simulink model "StateMachine"  (R2024a)
settings: Solver=ode4  StartTime=0.0  StopTime=10.0  FixedStep=1/1600  RelTol=1e-3
undefined symbols (not defined in the file): gains, initout, params, rates
libraries: simulink_extras x4, slpidlib x2, GT x1, aerolibasang x1
settings Model: Creator=igmso  LastModifiedBy=igmso

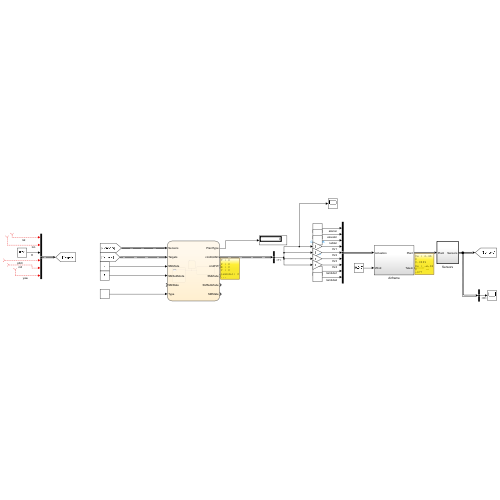
[thumbnail: Simulink's stored preview of the top-level diagram]
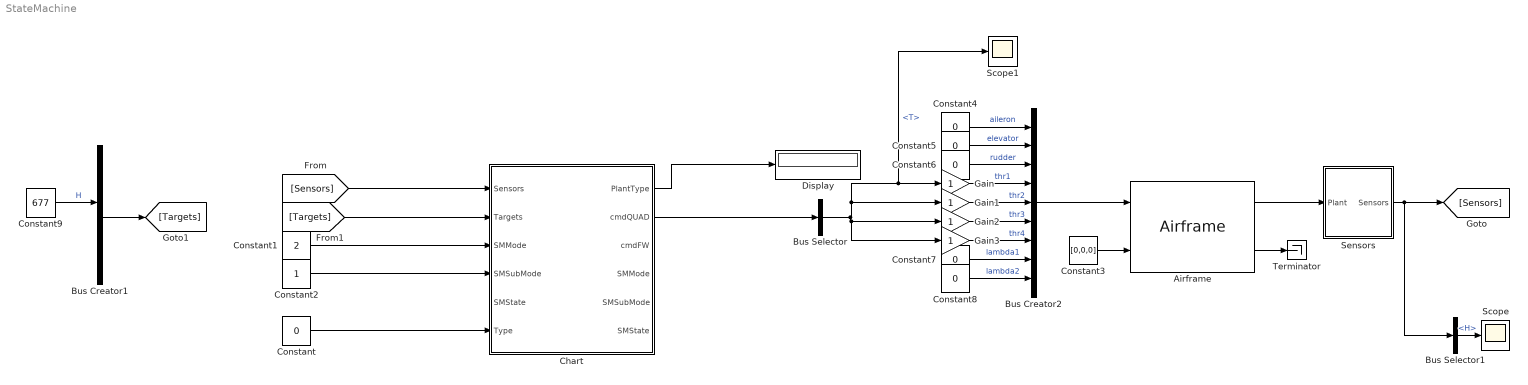
== system StateMachine ==
  Airframe : GT/Airframe  SystemSampleTime=-1  VariantActivationTime=update diagram  AllowFlexibleInterface=on  Latency=0  AutoFrameSizeCalculation=off
  Bus Creator1 : BusCreator  Inputs=6  OutDataTypeStr=Bus: targetsBus  NonVirtualBus=on
  Bus Creator2 : BusCreator  Inputs=9
  Bus Selector : BusSelector  OutputSignals=T
  Bus Selector1 : BusSelector  OutputSignals=H
  Chart : Stateflow chart  TreatAsAtomicUnit=on
      settings: PortSchema="{\"entries\":[{\"content\":{\"sides\":[{\"content\":{\"connectorIds\":[\"In1\",\"In2\",\"In3\",\"In4\",\"In5\",\"In6\"]},\"type\":\"ConnectorPlacement.EquallySpacedRectSide\",\"uuid\":\"c12811fb-1763-4b1f-8237-72373105f559\"},{\"content\":{\"connectorIds\":[\"Out1\",\"Out5\",\"Out6\",\"Out2\",\"Out3\",\"Out4\"],\"side\":\"RIGHT\"},\"type\":\"ConnectorPlacement.EquallySpacedRectSide\",\"uuid\":\"3712ff0d-cc13-4e2e-bfea-d52da842e5af\"},{\"content\":{\"side\":\"TOP\"},\"type\":\"ConnectorPlacement.EquallySpacedRectSide\",\"uuid\":\"ba161a25-7347-4103-889e-23a821fde0ef\"}]},\"type\":\"ConnectorPlacement.EquallySpacedConnector\",\"uuid\":\"8d874a7a-8fc0-4a11-bc61-1ae99cb768d4\"}],\"packageUris\":[\"http://schema.mathworks.com/mf0/Connector/R2020b\"],\"version\":\"1.0\"}"
  Constant{,4..8} (6 alike) : Constant  Value=0  SampleTime=-1
  Constant1 : Constant  Value=2  SampleTime=-1
  Constant2 : Constant  SampleTime=-1
  Constant3 : Constant  Value=[0,0,0]  SampleTime=-1
  Constant9 : Constant  Value=677  SampleTime=-1
  Display : Display
  Gain{,1..3} (4 alike) : Gain
  Scope : Scope
  Scope1 : Scope
  Sensors : Subsystem  TreatAsAtomicUnit=on  SystemSampleTime=1/400
  Terminator : Terminator
  wires:
  Constant/1 -> Chart/6(Type)
  Chart/1(PlantType) -> Display/1
  [Sensors] -> Chart/1(Sensors)
  Bus Creator1/1 -> [Targets]
  Constant9/1 -> Bus Creator1/3  "H"
  [Targets] -> Chart/2(Targets)
  Constant1/1 -> Chart/3("SMMode ")
  Constant2/1 -> Chart/4("SMSubMode ")
  Airframe/1 -> Sensors/1(Plant)
  Sensors/1(Sensors) -> Bus Selector1/1, [Sensors]
  Airframe/2 -> Terminator/1
  Constant3/1 -> Airframe/2
  Gain2/1 -> Bus Creator2/6  "thr3"
  Constant4/1 -> Bus Creator2/1  "aileron"
  Gain1/1 -> Bus Creator2/5  "thr2"
  Constant6/1 -> Bus Creator2/3  "rudder"
  Gain/1 -> Bus Creator2/4  "thr1"
  Constant8/1 -> Bus Creator2/9  "lambda2"
  Gain3/1 -> Bus Creator2/7  "thr4"
  Constant7/1 -> Bus Creator2/8  "lambda1"
  Constant5/1 -> Bus Creator2/2  "elevator"
  Bus Creator2/1 -> Airframe/1
  Chart/5(cmdQUAD) -> Bus Selector/1
  Bus Selector/1 -> Gain3/1, Gain2/1, Gain1/1, Scope1/1, Gain/1  "<T>"
  ? -> Bus Creator1/1  "lat"
  ? -> Bus Creator1/2  "lon"
  ? -> Bus Creator1/4  "pitch"
  ? -> Bus Creator1/5  "roll"
  ? -> Bus Creator1/6  "yaw"
  Bus Selector1/1 -> Scope/1  "<H>"

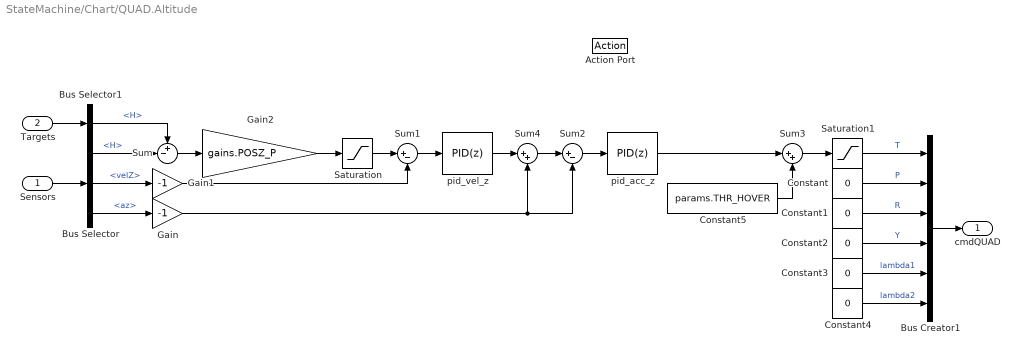
== system StateMachine/Chart/QUAD.Altitude ==
  Sensors : Inport  OutDataTypeStr=Bus: sensorsBus
  Targets : Inport  Port=2  OutDataTypeStr=Bus: targetsBus
  Action Port : ActionPort
      settings: CopyFcn=Stateflow.SLINSF.SimulinkMan.removeBlockPreDeleteFcn  PreDeleteFcn=Stateflow.SLINSF.SimulinkMan.unsafePredeleteFcn
  Bus Creator1 : BusCreator  Inputs=6  OutDataTypeStr=Bus: cmdQUADBus  NonVirtualBus=on
  Bus Selector : BusSelector  OutputSignals=H,velZ,az
  Bus Selector1 : BusSelector  OutputSignals=H
  Constant{,1..4} (5 alike) : Constant  Value=0  SampleTime=-1
  Constant5 : Constant  Value=params.THR_HOVER
  Gain : Gain  Gain=-1
  Gain1 : Gain  Gain=-1
  Gain2 : Gain  Gain=gains.POSZ_P
  Saturation : Saturate  UpperLimit=1  LowerLimit=-1
  Saturation1 : Saturate  UpperLimit=1  LowerLimit=0
  Sum : Sum  Inputs=+-|
  Sum1 : Sum  Inputs=|+-
  Sum2 : Sum  Inputs=|+-
  Sum3 : Sum  Inputs=|++
  Sum4 : Sum  Inputs=|++
  pid_acc_z : slpidlib/PID Controller  Controller=PID  Form=Parallel  TimeDomain=Discrete-time  UseExternalTs=off  SampleTime=rates.Altitude  IntegratorMethod=Forward Euler  FilterMethod=Forward Euler  ControllerParametersSource=internal  P=gains.ACCZ_P  I=gains.ACCZ_I  UseKiTs=on  D=gains.ACCZ_D  UseExternalDerivativeSource=off  N=gains.ACCZ_FF  UseFilter=on  TunerSelectOption=Transfer Function Based (PID Tuner App)  InitialConditionSource=internal  InitialConditionForIntegrator=0  InitialConditionForFilter=0  DifferentiatorICPrevScaledInput=0  ExternalReset=none  TrackingMode=off  Kt=1  LimitOutput=off  SatLimitsSource=internal  UpperSaturationLimit=params.CLIMB_MAX  LowerSaturationLimit=-params.SINK_MAX  LinearizeAsGain=on  AntiWindupMode=clamping  Kb=1  LimitIntegrator=on  UpperIntegratorSaturationLimit=gains.VELZ_IMAX  LowerIntegratorSaturationLimit=-gains.VELZ_IMAX  POutMin=[]  POutMax=[]  IOutMin=[]  IOutMax=[]  DOutMin=[]  DOutMax=[]  NOutMin=[]  NOutMax=[]  SumOutMin=[]  SumOutMax=[]  SaturationOutMin=[]  SaturationOutMax=[]  PParamMin=[]  PParamMax=[]  IParamMin=[]  IParamMax=[]  DParamMin=[]  DParamMax=[]  NParamMin=[]  NParamMax=[]  KbParamMin=[]  KbParamMax=[]  KtParamMin=[]  KtParamMax=[]  KbOutMin=[]  KbOutMax=[]  KtOutMin=[]  KtOutMax=[]  IntegratorOutMin=[]  IntegratorOutMax=[]  FilterOutMin=[]  FilterOutMax=[]  SumI1OutMin=[]  SumI1OutMax=[]  SumI2OutMin=[]  SumI2OutMax=[]  SumI3OutMin=[]  SumI3OutMax=[]  SumI4OutMin=[]  SumI4OutMax=[]  SumDOutMin=[]  SumDOutMax=[]  DifferentiatorOutMin=[]  DifferentiatorOutMax=[]  FilterDiffOutCoefMin=[]  FilterDiffOutCoefMax=[]  ReciprocalOutMin=[]  ReciprocalOutMax=[]  SumDenOutMin=[]  SumDenOutMax=[]  SumNumOutMin=[]  SumNumOutMax=[]  DivideOutMin=[]  DivideOutMax=[]  UdiffTsProdOutMin=[]  UdiffTsProdOutMax=[]  NTsProdOutMin=[]  NTsProdOutMax=[]  UintegralTsProdOutMin=[]  UintegralTsProdOutMax=[]  UngainTsProdOutMin=[]  UngainTsProdOutMax=[]  ClampingZeroOutDataTypeStr=Inherit: Inherit via back propagation  ClampingZeroOutMin=[]  ClampingZeroOutMax=[]  FilterDenConstantOutDataTypeStr=Inherit: Inherit via back propagation  FilterDenConstantOutMin=[]  FilterDenConstantOutMax=[]  PCopyOutDataTypeStr=Inherit: Inherit via back propagation  PCopyOutMin=[]  PCopyOutMax=[]  NCopyOutDataTypeStr=Inherit: Inherit via back propagation  NCopyOutMin=[]  NCopyOutMax=[]  IntegratorContinuousStateAttributes=''  IntegratorStateIdentifier="\"VELZ\""  IntegratorStateMustResolveToSignalObject=off  IntegratorRTWStateStorageClass=Auto  FilterContinuousStateAttributes=''  FilterStateIdentifier="\"VELZ\""  FilterStateMustResolveToSignalObject=off  FilterRTWStateStorageClass=Auto  ParallelPVariant=InternalParameters  IdealPVariant=Disabled  IVariant=InternalParameters  DVariant=InternalParameters  IntegratorVariant=Discrete  SatVariant=Disabled  AWVariant=Passthrough  PCopyVariant=Disabled  TRVariant=Disabled  FdbkBlocksVariant=Forward  IdealPFdbkVariant=Disabled  SatFdbkVariant=Disabled  DerivativeFilterVariant=ForwardEulerFilter  NVariant=InternalParameters  NCopyVariant=Disabled  FilterICVariant=InternalICsFilter  IntegratorICVariant=InternalICs  ExternalResetVariant=Disabled  TRSumVariant=Passthrough  SumFdbkVariant=Disabled  SumVariant=Sum_PID  TsampFilterVariant=InternalTs  TsampNgainVariant=Passthrough  TsampIntegralVariant=Disabled_SignalSpec  ExternalSaturationOutDataTypeStr=Inherit: Same as second input  DerivativeSourceVariant=ErrorSignal
  pid_vel_z : slpidlib/PID Controller  Controller=PID  Form=Parallel  TimeDomain=Discrete-time  UseExternalTs=off  SampleTime=rates.Altitude  IntegratorMethod=Forward Euler  FilterMethod=Forward Euler  ControllerParametersSource=internal  P=gains.VELZ_P  I=gains.VELZ_I  UseKiTs=on  D=gains.VELZ_D  UseExternalDerivativeSource=off  N=gains.VELZ_FF  UseFilter=on  TunerSelectOption=Transfer Function Based (PID Tuner App)  InitialConditionSource=internal  InitialConditionForIntegrator=0  InitialConditionForFilter=0  DifferentiatorICPrevScaledInput=0  ExternalReset=none  TrackingMode=off  Kt=1  LimitOutput=off  SatLimitsSource=internal  UpperSaturationLimit=params.CLIMB_MAX  LowerSaturationLimit=-params.SINK_MAX  LinearizeAsGain=on  AntiWindupMode=clamping  Kb=1  LimitIntegrator=on  UpperIntegratorSaturationLimit=gains.VELZ_IMAX  LowerIntegratorSaturationLimit=-gains.VELZ_IMAX  POutMin=[]  POutMax=[]  IOutMin=[]  IOutMax=[]  DOutMin=[]  DOutMax=[]  NOutMin=[]  NOutMax=[]  SumOutMin=[]  SumOutMax=[]  SaturationOutMin=[]  SaturationOutMax=[]  PParamMin=[]  PParamMax=[]  IParamMin=[]  IParamMax=[]  DParamMin=[]  DParamMax=[]  NParamMin=[]  NParamMax=[]  KbParamMin=[]  KbParamMax=[]  KtParamMin=[]  KtParamMax=[]  KbOutMin=[]  KbOutMax=[]  KtOutMin=[]  KtOutMax=[]  IntegratorOutMin=[]  IntegratorOutMax=[]  FilterOutMin=[]  FilterOutMax=[]  SumI1OutMin=[]  SumI1OutMax=[]  SumI2OutMin=[]  SumI2OutMax=[]  SumI3OutMin=[]  SumI3OutMax=[]  SumI4OutMin=[]  SumI4OutMax=[]  SumDOutMin=[]  SumDOutMax=[]  DifferentiatorOutMin=[]  DifferentiatorOutMax=[]  FilterDiffOutCoefMin=[]  FilterDiffOutCoefMax=[]  ReciprocalOutMin=[]  ReciprocalOutMax=[]  SumDenOutMin=[]  SumDenOutMax=[]  SumNumOutMin=[]  SumNumOutMax=[]  DivideOutMin=[]  DivideOutMax=[]  UdiffTsProdOutMin=[]  UdiffTsProdOutMax=[]  NTsProdOutMin=[]  NTsProdOutMax=[]  UintegralTsProdOutMin=[]  UintegralTsProdOutMax=[]  UngainTsProdOutMin=[]  UngainTsProdOutMax=[]  ClampingZeroOutDataTypeStr=Inherit: Inherit via back propagation  ClampingZeroOutMin=[]  ClampingZeroOutMax=[]  FilterDenConstantOutDataTypeStr=Inherit: Inherit via back propagation  FilterDenConstantOutMin=[]  FilterDenConstantOutMax=[]  PCopyOutDataTypeStr=Inherit: Inherit via back propagation  PCopyOutMin=[]  PCopyOutMax=[]  NCopyOutDataTypeStr=Inherit: Inherit via back propagation  NCopyOutMin=[]  NCopyOutMax=[]  IntegratorContinuousStateAttributes=''  IntegratorStateIdentifier="\"VELZ\""  IntegratorStateMustResolveToSignalObject=off  IntegratorRTWStateStorageClass=Auto  FilterContinuousStateAttributes=''  FilterStateIdentifier="\"VELZ\""  FilterStateMustResolveToSignalObject=off  FilterRTWStateStorageClass=Auto  ParallelPVariant=InternalParameters  IdealPVariant=Disabled  IVariant=InternalParameters  DVariant=InternalParameters  IntegratorVariant=Discrete  SatVariant=Disabled  AWVariant=Passthrough  PCopyVariant=Disabled  TRVariant=Disabled  FdbkBlocksVariant=Forward  IdealPFdbkVariant=Disabled  SatFdbkVariant=Disabled  DerivativeFilterVariant=ForwardEulerFilter  NVariant=InternalParameters  NCopyVariant=Disabled  FilterICVariant=InternalICsFilter  IntegratorICVariant=InternalICs  ExternalResetVariant=Disabled  TRSumVariant=Passthrough  SumFdbkVariant=Disabled  SumVariant=Sum_PID  TsampFilterVariant=InternalTs  TsampNgainVariant=Passthrough  TsampIntegralVariant=Disabled_SignalSpec  ExternalSaturationOutDataTypeStr=Inherit: Same as second input  DerivativeSourceVariant=ErrorSignal
  cmdQUAD : Outport  OutDataTypeStr=Bus: cmdQUADBus
  wires:
  Sensors/1 -> Bus Selector/1
  Bus Selector/3 -> Gain/1  "<az>"
  Bus Selector/2 -> Gain1/1  "<velZ>"
  Bus Selector/1 -> Sum/2  "<H>"
  Bus Selector1/1 -> Sum/1  "<H>"
  Targets/1 -> Bus Selector1/1
  Sum/1 -> Gain2/1
  Gain2/1 -> Saturation/1
  Gain1/1 -> Sum1/2
  Sum1/1 -> pid_vel_z/1
  pid_vel_z/1 -> Sum4/1
  Gain/1 -> Sum4/2, Sum2/2
  Sum2/1 -> pid_acc_z/1
  Saturation/1 -> Sum1/1
  Saturation1/1 -> Bus Creator1/1  "T"
  pid_acc_z/1 -> Sum3/1
  Constant/1 -> Bus Creator1/2  "P"
  Constant1/1 -> Bus Creator1/3  "R"
  Constant2/1 -> Bus Creator1/4  "Y"
  Constant3/1 -> Bus Creator1/5  "lambda1"
  Constant4/1 -> Bus Creator1/6  "lambda2"
  Bus Creator1/1 -> cmdQUAD/1
  Sum3/1 -> Saturation1/1
  Constant5/1 -> Sum3/2
  Sum4/1 -> Sum2/1

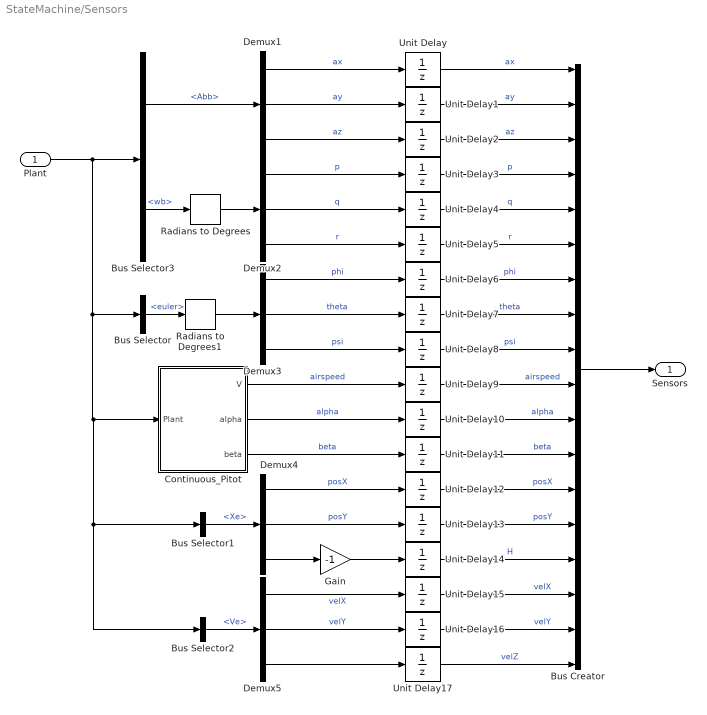
== system StateMachine/Sensors ==
  Plant : Inport
  Bus Selector : BusSelector  OutputSignals=euler
  Bus Selector1 : BusSelector  OutputSignals=Xe
  Bus Selector2 : BusSelector  OutputSignals=Ve
  Bus Selector3 : BusSelector  OutputSignals=Abb,wb
  Bus Creator : BusCreator  Inputs=18  OutDataTypeStr=Bus: sensorsBus  NonVirtualBus=on
  Continuous_Pitot : Subsystem
  Demux{1..5} (5 alike) : Demux  Outputs=3
  Gain : Gain  Gain=-1
  Radians to Degrees : simulink_extras/Transformations/Radians to Degrees
  Radians to Degrees1 : simulink_extras/Transformations/Radians to Degrees
  Unit Delay : UnitDelay  InitialCondition=initout(1)  SampleTime=-1  HasFrameUpgradeWarning=on
  Unit Delay1 : UnitDelay  InitialCondition=initout(2)  SampleTime=-1  HasFrameUpgradeWarning=on
  Unit Delay10 : UnitDelay  InitialCondition=initout(11)  SampleTime=-1  HasFrameUpgradeWarning=on
  Unit Delay11 : UnitDelay  InitialCondition=initout(12)  SampleTime=-1  HasFrameUpgradeWarning=on
  Unit Delay12 : UnitDelay  InitialCondition=initout(13)  SampleTime=-1  HasFrameUpgradeWarning=on
  Unit Delay13 : UnitDelay  InitialCondition=initout(14)  SampleTime=-1  HasFrameUpgradeWarning=on
  Unit Delay14 : UnitDelay  InitialCondition=initout(15)  SampleTime=-1  HasFrameUpgradeWarning=on
  Unit Delay15 : UnitDelay  InitialCondition=initout(16)  SampleTime=-1  HasFrameUpgradeWarning=on
  Unit Delay16 : UnitDelay  InitialCondition=initout(17)  SampleTime=-1  HasFrameUpgradeWarning=on
  Unit Delay17 : UnitDelay  InitialCondition=initout(18)  SampleTime=-1  HasFrameUpgradeWarning=on
  Unit Delay2 : UnitDelay  InitialCondition=initout(3)  SampleTime=-1  HasFrameUpgradeWarning=on
  Unit Delay3 : UnitDelay  InitialCondition=initout(4)  SampleTime=-1  HasFrameUpgradeWarning=on
  Unit Delay4 : UnitDelay  InitialCondition=initout(5)  SampleTime=-1  HasFrameUpgradeWarning=on
  Unit Delay5 : UnitDelay  InitialCondition=initout(6)  SampleTime=-1  HasFrameUpgradeWarning=on
  Unit Delay6 : UnitDelay  InitialCondition=initout(7)  SampleTime=-1  HasFrameUpgradeWarning=on
  Unit Delay7 : UnitDelay  InitialCondition=initout(8)  SampleTime=-1  HasFrameUpgradeWarning=on
  Unit Delay8 : UnitDelay  InitialCondition=initout(9)  SampleTime=-1  HasFrameUpgradeWarning=on
  Unit Delay9 : UnitDelay  InitialCondition=initout(10)  SampleTime=-1  HasFrameUpgradeWarning=on
  Sensors : Outport  OutDataTypeStr=Bus: sensorsBus
  wires:
  Unit Delay2/1 -> Bus Creator/3  "az"
  Unit Delay1/1 -> Bus Creator/2  "ay"
  Unit Delay/1 -> Bus Creator/1  "ax"
  Bus Selector3/1 -> Demux1/1  "<Abb>"
  Bus Selector3/2 -> Radians to Degrees/1  "<wb>"
  Unit Delay3/1 -> Bus Creator/4  "p"
  Unit Delay4/1 -> Bus Creator/5  "q"
  Unit Delay5/1 -> Bus Creator/6  "r"
  Bus Selector/1 -> Radians to Degrees1/1  "<euler>"
  Unit Delay6/1 -> Bus Creator/7  "phi"
  Unit Delay7/1 -> Bus Creator/8  "theta"
  Unit Delay8/1 -> Bus Creator/9  "psi"
  Bus Selector1/1 -> Demux4/1  "<Xe>"
  Bus Creator/1 -> Sensors/1
  Bus Selector2/1 -> Demux5/1  "<Ve>"
  Radians to Degrees/1 -> Demux2/1
  Radians to Degrees1/1 -> Demux3/1
  Unit Delay9/1 -> Bus Creator/10  "airspeed"
  Unit Delay10/1 -> Bus Creator/11  "alpha"
  Unit Delay11/1 -> Bus Creator/12  "beta"
  Unit Delay12/1 -> Bus Creator/13  "posX"
  Unit Delay13/1 -> Bus Creator/14  "posY"
  Unit Delay14/1 -> Bus Creator/15  "H"
  Unit Delay15/1 -> Bus Creator/16  "velX"
  Unit Delay16/1 -> Bus Creator/17  "velY"
  Unit Delay17/1 -> Bus Creator/18  "velZ"
  Continuous_Pitot/1(V) -> Unit Delay9/1  "airspeed"
  Continuous_Pitot/2(alpha) -> Unit Delay10/1  "alpha"
  Continuous_Pitot/3(beta) -> Unit Delay11/1  "beta"
  Demux1/1 -> Unit Delay/1  "ax"
  Demux1/2 -> Unit Delay1/1  "ay"
  Demux1/3 -> Unit Delay2/1  "az"
  Demux2/1 -> Unit Delay3/1  "p"
  Demux2/2 -> Unit Delay4/1  "q"
  Demux2/3 -> Unit Delay5/1  "r"
  Demux3/1 -> Unit Delay6/1  "phi"
  Demux3/2 -> Unit Delay7/1  "theta"
  Demux3/3 -> Unit Delay8/1  "psi"
  Demux4/2 -> Unit Delay13/1  "posY"
  Demux4/3 -> Gain/1
  Demux4/1 -> Unit Delay12/1  "posX"
  Gain/1 -> Unit Delay14/1
  Demux5/1 -> Unit Delay15/1  "velX"
  Demux5/2 -> Unit Delay16/1  "velY"
  Demux5/3 -> Unit Delay17/1
  Plant/1 -> Bus Selector2/1, Bus Selector1/1, Continuous_Pitot/1(Plant), Bus Selector/1, Bus Selector3/1

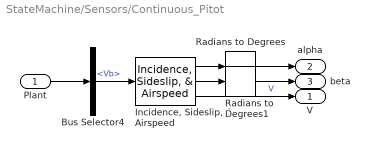
== system StateMachine/Sensors/Continuous_Pitot ==
  Plant : Inport
  Bus Selector4 : BusSelector  OutputSignals=Vb
  "Incidence, Sideslip, & Airspeed" : aerolibasang/Incidence, Sideslip, & Airspeed
  Radians to Degrees : simulink_extras/Transformations/Radians to Degrees
  Radians to Degrees1 : simulink_extras/Transformations/Radians to Degrees
  V : Outport
  alpha : Outport  Port=2
  beta : Outport  Port=3
  wires:
  Bus Selector4/1 -> "Incidence, Sideslip, & Airspeed"/1  "<Vb>"
  "Incidence, Sideslip, & Airspeed"/1 -> Radians to Degrees/1
  Plant/1 -> Bus Selector4/1
  "Incidence, Sideslip, & Airspeed"/3 -> V/1  "V"
  "Incidence, Sideslip, & Airspeed"/2 -> Radians to Degrees1/1
  Radians to Degrees/1 -> alpha/1
  Radians to Degrees1/1 -> beta/1

== stateflow chart StateMachine/Chart ==
  settings: updateMethod=DISCRETE  sampleTime=1/400
  state Start
    en:
    PlantType = Type;
    SMMode = 0;
    SMSubMode = 0;
    SMState = 0;
    cmdQUAD.T = THR_HOVER;
    cmdQUAD.P = 0;
    cmdQUAD.R = 0;
    cmdQUAD.Y = 0;
    cmdQUAD.lambda1 = 0;
    cmdQUAD.lambda2 = 0;
    cmdFW.aileron = 0;
    cmdFW.elevator = 0;
    cmdFW.rudder = 0;
    cmdFW.throttle = 0;
    cmdFW.lambda1 = 0;
    cmdFW.lambda2 = 0;
  state FixedWing
  state QUAD
    state Altitude
    QUAD -> Altitude : [SMMode == 2  && SMSubMode == 1]
        | {SMMode = 2, SMSubMode = 1,
        |  cmdFW.aileron = 0, cmdFW.elevator = 0,
        | cmdFW.rudder = 0, cmdFW.throttle = 0,
        | cmdFW.lambda1 = 0, cmdFW.lambda2 = 0}
  (default) -> Start
  Start -> (junction 49)
  (junction 49) -> QUAD [order 1] : [(PlantType == 0)]
  (junction 49) -> FixedWing [order 2] : [(PlantType == 0)]
  data: sf_internal_action_state_placeholder_data local double size=1 =0; Sensors input Bus: sensorsBus; Targets input Bus: targetsBus; SMMode input; SMSubMode input; SMState input; PlantType output; SMMode output; SMSubMode output; SMState output; Type input; cmdQUAD output Bus: cmdQUADBus; cmdFW output Bus: cmdFWBus; THR_HOVER constant double =params.THR_HOVER
